simulink model "Energy_based_CBF_shishir"  (R2023b)
settings: Solver=ode5  StartTime=0.0  StopTime=4  FixedStep=0.00001  RelTol=1e-3
settings Model: Creator=amaiani  LastModifiedBy=amaiani

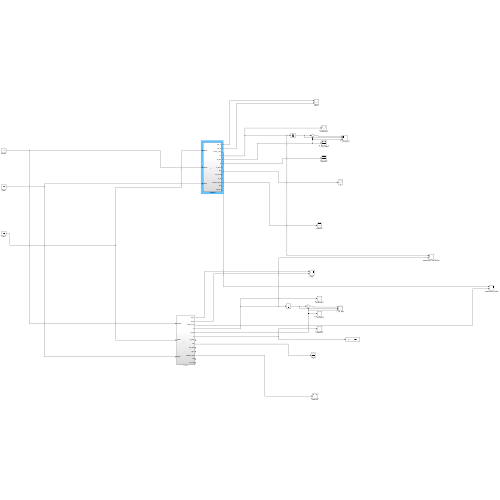
[thumbnail: Simulink's stored preview of the top-level diagram]
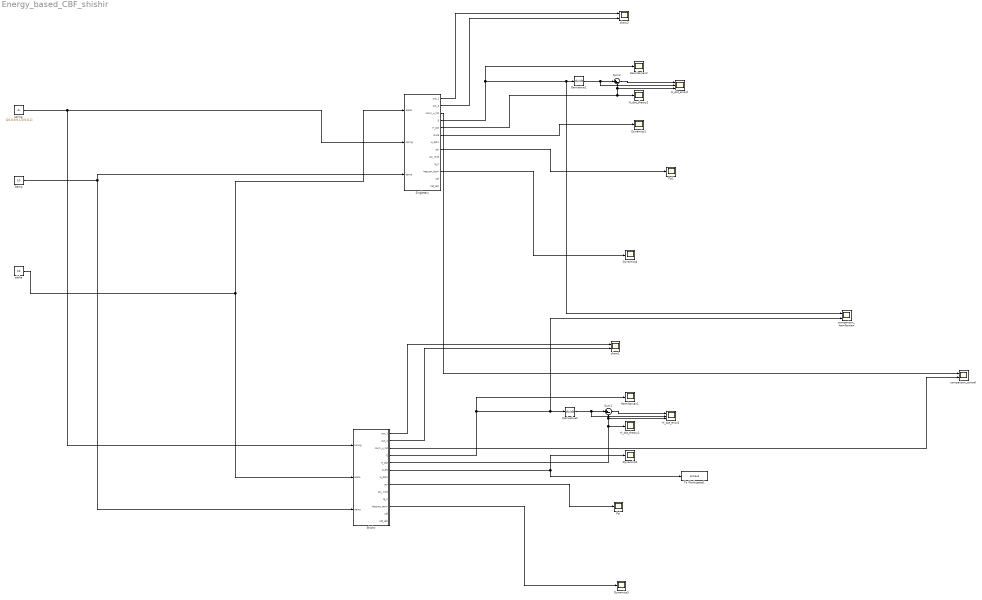
== system Energy_based_CBF_shishir ==
  Damp : Constant  Value=10
  Derivative1 : Derivative
  Derivative2 : Derivative
  Dynamics{1..4} (4 alike) : Scope
  H_dot_error1 : Scope  NumInputPorts=3
  H_dot_error2 : Scope  NumInputPorts=3
  H_dot_theory1 : Scope
  H_dot_theory2 : Scope
  Hamiltonian1 : Scope
  Hamiltonian2 : Scope
  Psi : Scope
  Psi1 : Scope
  Shishir : Subsystem
  Singletary : Subsystem
  Sum1 : Sum  Inputs=|+-
  Sum2 : Sum  Inputs=|+-
  To Workspace1 : ToWorkspace  VariableName=simout  SampleTime=-1
  alpha : Constant  Value=10
  comparison_control : Scope  NumInputPorts=2
  comparison_hamiltonian : Scope  NumInputPorts=2
  skew1 : Scope  NumInputPorts=2
  skew2 : Scope  NumInputPorts=2
  spring : Constant  Value=[10,0,0;0,1,0;0,0,1]
  wires:
  Derivative2/1 -> H_dot_error1/2, Sum1/1
  Sum1/1 -> H_dot_error1/1
  alpha/1 -> Singletary/1(alpha), Shishir/2(alpha)
  Shishir/5(H_dot) -> H_dot_theory1/1, H_dot_error1/3, Sum1/2
  Shishir/4(E) -> Derivative2/1, comparison_hamiltonian/2, Hamiltonian1/1
  Shishir/1(out_1) -> skew1/1
  Shishir/2(out_2) -> skew1/2
  Shishir/3(norm_u_tot) -> comparison_control/2
  Shishir/6(Out6) -> Dynamics2/1, To Workspace1/1
  Shishir/11(hessian_term) -> Dynamics3/1
  Derivative1/1 -> H_dot_error2/2, Sum2/1
  Singletary/1(out_1) -> skew2/1
  Singletary/5(H_dot) -> H_dot_theory2/1, H_dot_error2/3, Sum2/2
  Damp/1 -> Singletary/3(damp), Shishir/3(damp)
  Singletary/2(out_2) -> skew2/2
  Singletary/4(E) -> comparison_hamiltonian/1, Derivative1/1, Hamiltonian2/1
  Sum2/1 -> H_dot_error2/1
  Singletary/3(norm_u_tot) -> comparison_control/1
  Singletary/11(hessian_term) -> Dynamics4/1
  Singletary/6(Out6) -> Dynamics1/1
  spring/1 -> Singletary/2(spring), Shishir/1(spring)
  Shishir/8(psi) -> Psi/1
  Singletary/8(psi) -> Psi1/1

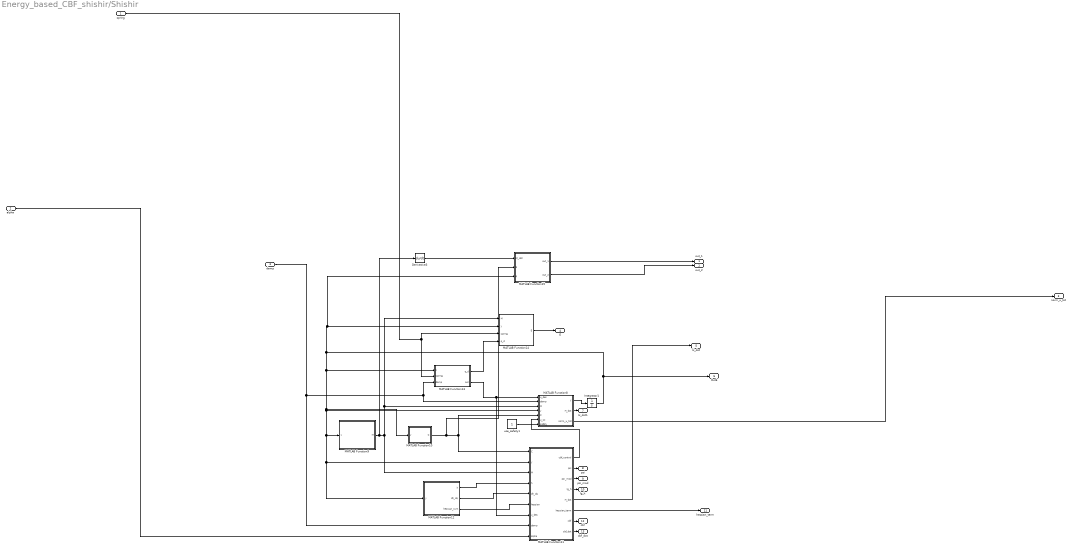
== system Energy_based_CBF_shishir/Shishir ==
  spring : Inport
  alpha : Inport  Port=2
  damp : Inport  Port=3
  Derivative3 : Derivative
  Integrator1 : Integrator  InitialCondition=[0;0;0;0;0;0]
  MATLAB Function10 : MATLAB Function  StartFcn=|  TreatAsAtomicUnit=on
      | % Define numerical values for the parameters
      | xc = 2.5;
      | yc = 2;
      | r = 1;
      | gamma = 2;
      | alpha = 20;
      | 
      | 
      | m1 = 1;
      | m2 = 1;
      | m3 = 1;
      | 
      | 
      | l1 = 1;
      | l2 = 1;
      | l3 = 1;
  MATLAB Function11 : MATLAB Function  TreatAsAtomicUnit=on
  MATLAB Function12 : MATLAB Function  TreatAsAtomicUnit=on
  MATLAB Function13 : MATLAB Function  TreatAsAtomicUnit=on
  MATLAB Function14 : MATLAB Function  TreatAsAtomicUnit=on
  MATLAB Function15 : MATLAB Function  StartFcn=|  TreatAsAtomicUnit=on
      | % Define numerical values for the parameters
      | xc = 2.5;
      | yc = 2;
      | r = 1;
      | gamma = 2;
      | alpha = 20;
      | 
      | 
      | m1 = 1;
      | m2 = 1;
      | m3 = 1;
      | 
      | 
      | l1 = 1;
      | l2 = 1;
      | l3 = 1;
  MATLAB Function8 : MATLAB Function  TreatAsAtomicUnit=on
  MATLAB Function9 : MATLAB Function  StartFcn=|  TreatAsAtomicUnit=on
      | % Define numerical values for the parameters
      | xc = 2.5;
      | yc = 2;
      | r = 1;
      | gamma = 2;
      | alpha = 20;
      | 
      | 
      | m1 = 1;
      | m2 = 1;
      | m3 = 1;
      | 
      | 
      | l1 = 1;
      | l2 = 1;
      | l3 = 1;
  use_safety1 : Constant
  out_1 : Outport
  out_2 : Outport  Port=2
  norm_u_tot : Outport  Port=3
  E : Outport  Port=4
  H_dot : Outport  Port=5
  Out6 : Outport  Port=6
  H_dot1 : Outport  Port=7
  psi : Outport  Port=8
  psi_mod : Outport  Port=9
  lg_h : Outport  Port=10
  hessian_term : Outport  Port=11
  cbf : Outport  Port=12
  cbf_dot : Outport  Port=13
  wires:
  MATLAB Function11/2(psi) -> psi/1
  MATLAB Function11/4(lg_h) -> lg_h/1
  MATLAB Function11/7(cbf) -> cbf/1
  MATLAB Function8/2(H_dot) -> H_dot1/1
  MATLAB Function11/5(H_dot) -> H_dot/1
  MATLAB Function11/6(hessian_term) -> hessian_term/1
  MATLAB Function14/1(E) -> E/1
  MATLAB Function8/3(norm_u_tot) -> norm_u_tot/1
  MATLAB Function12/3(hessian_sym) -> MATLAB Function11/6(hessian)
  Derivative3/1 -> MATLAB Function15/1(M_dot)
  MATLAB Function12/1(h) -> MATLAB Function11/4(h)
  MATLAB Function8/1(y) -> Integrator1/1
  MATLAB Function11/3(psi_mod) -> psi_mod/1
  alpha/1 -> MATLAB Function11/9(alpha)
  spring/1 -> MATLAB Function13/2(spring), MATLAB Function14/3(spring)
  MATLAB Function10/1(C) -> MATLAB Function8/5(C), MATLAB Function11/1(C), MATLAB Function15/2(S)
  MATLAB Function13/1(q_d) -> MATLAB Function14/4(q_d)
  MATLAB Function11/1(cbf_control) -> MATLAB Function8/6(u_sc)
  MATLAB Function15/2(out_2) -> out_2/1
  Integrator1/1 -> Out6/1, MATLAB Function15/3(q), MATLAB Function14/2(y), MATLAB Function13/1(y), MATLAB Function10/1(y), MATLAB Function12/1(y), MATLAB Function11/2(y), MATLAB Function9/1(y), MATLAB Function8/4("y ")
  MATLAB Function15/1(out_1) -> out_1/1
  damp/1 -> MATLAB Function11/8(damp), MATLAB Function8/2(damp), MATLAB Function13/3(damp)
  MATLAB Function12/2(dh_dq) -> MATLAB Function11/5(dh_dq)
  MATLAB Function13/2(out) -> MATLAB Function11/7(u_des), MATLAB Function8/1(u_des)
  MATLAB Function11/8(cbf_dot) -> cbf_dot/1
  use_safety1/1 -> MATLAB Function8/7(safety)
  MATLAB Function9/1(M) -> Derivative3/1, MATLAB Function14/1(M), MATLAB Function8/3(M), MATLAB Function11/3(M)

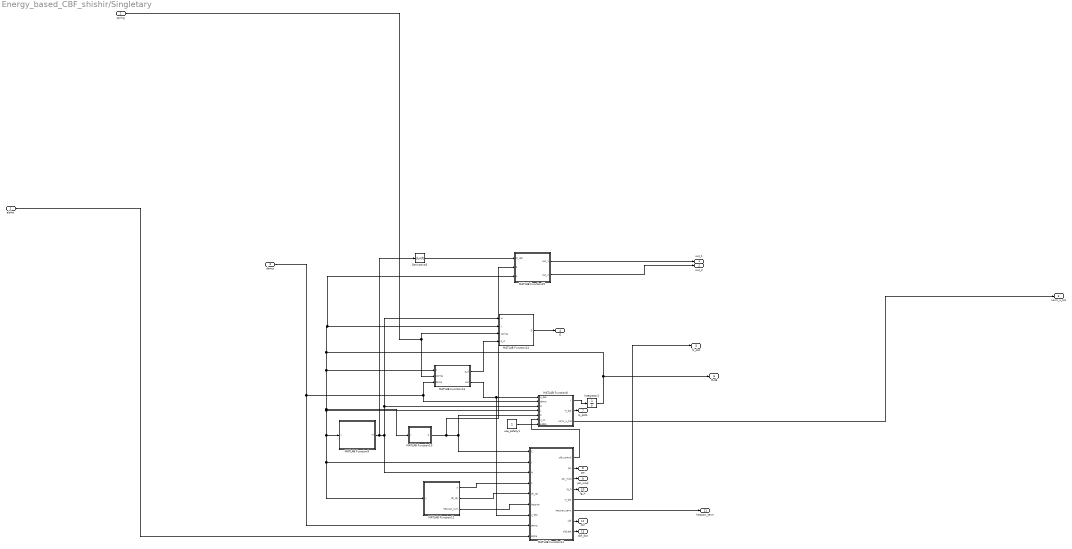
== system Energy_based_CBF_shishir/Singletary ==
  alpha : Inport
  spring : Inport  Port=2
  damp : Inport  Port=3
  Derivative3 : Derivative
  Integrator1 : Integrator  InitialCondition=[0;0;0;0;0;0]
  MATLAB Function10 : MATLAB Function  StartFcn=|  TreatAsAtomicUnit=on
      | % Define numerical values for the parameters
      | xc = 2.5;
      | yc = 2;
      | r = 1;
      | gamma = 2;
      | alpha = 20;
      | 
      | 
      | m1 = 1;
      | m2 = 1;
      | m3 = 1;
      | 
      | 
      | l1 = 1;
      | l2 = 1;
      | l3 = 1;
  MATLAB Function11 : MATLAB Function  TreatAsAtomicUnit=on
  MATLAB Function12 : MATLAB Function  TreatAsAtomicUnit=on
  MATLAB Function13 : MATLAB Function  TreatAsAtomicUnit=on
  MATLAB Function14 : MATLAB Function  TreatAsAtomicUnit=on
  MATLAB Function15 : MATLAB Function  StartFcn=|  TreatAsAtomicUnit=on
      | % Define numerical values for the parameters
      | xc = 2.5;
      | yc = 2;
      | r = 1;
      | gamma = 2;
      | alpha = 20;
      | 
      | 
      | m1 = 1;
      | m2 = 1;
      | m3 = 1;
      | 
      | 
      | l1 = 1;
      | l2 = 1;
      | l3 = 1;
  MATLAB Function8 : MATLAB Function  TreatAsAtomicUnit=on
  MATLAB Function9 : MATLAB Function  StartFcn=|  TreatAsAtomicUnit=on
      | % Define numerical values for the parameters
      | xc = 2.5;
      | yc = 2;
      | r = 1;
      | gamma = 2;
      | alpha = 20;
      | 
      | 
      | m1 = 1;
      | m2 = 1;
      | m3 = 1;
      | 
      | 
      | l1 = 1;
      | l2 = 1;
      | l3 = 1;
  use_safety1 : Constant
  out_1 : Outport
  out_2 : Outport  Port=2
  norm_u_tot : Outport  Port=3
  E : Outport  Port=4
  H_dot : Outport  Port=5
  Out6 : Outport  Port=6
  H_dot1 : Outport  Port=7
  psi : Outport  Port=8
  psi_mod : Outport  Port=9
  lg_h : Outport  Port=10
  hessian_term : Outport  Port=11
  cbf : Outport  Port=12
  cbf_dot : Outport  Port=13
  wires:
  MATLAB Function11/2(psi) -> psi/1
  MATLAB Function11/4(lg_h) -> lg_h/1
  MATLAB Function11/7(cbf) -> cbf/1
  MATLAB Function8/2(H_dot) -> H_dot1/1
  MATLAB Function11/5(H_dot) -> H_dot/1
  MATLAB Function11/6(hessian_term) -> hessian_term/1
  MATLAB Function14/1(E) -> E/1
  MATLAB Function8/3(norm_u_tot) -> norm_u_tot/1
  MATLAB Function12/3(hessian_sym) -> MATLAB Function11/6(hessian)
  Derivative3/1 -> MATLAB Function15/1(M_dot)
  MATLAB Function12/1(h) -> MATLAB Function11/4(h)
  MATLAB Function8/1(y) -> Integrator1/1
  MATLAB Function11/3(psi_mod) -> psi_mod/1
  alpha/1 -> MATLAB Function11/9(alpha)
  spring/1 -> MATLAB Function13/2(spring), MATLAB Function14/3(spring)
  MATLAB Function10/1(C) -> MATLAB Function8/5(C), MATLAB Function11/1(C), MATLAB Function15/2(S)
  MATLAB Function13/1(q_d) -> MATLAB Function14/4(q_d)
  MATLAB Function11/1(cbf_control) -> MATLAB Function8/6(u_sc)
  MATLAB Function15/2(out_2) -> out_2/1
  Integrator1/1 -> Out6/1, MATLAB Function15/3(q), MATLAB Function14/2(y), MATLAB Function13/1(y), MATLAB Function10/1(y), MATLAB Function12/1(y), MATLAB Function11/2(y), MATLAB Function9/1(y), MATLAB Function8/4("y ")
  MATLAB Function15/1(out_1) -> out_1/1
  damp/1 -> MATLAB Function11/8(damp), MATLAB Function8/2(damp), MATLAB Function13/3(damp)
  MATLAB Function12/2(dh_dq) -> MATLAB Function11/5(dh_dq)
  MATLAB Function13/2(out) -> MATLAB Function11/7(u_des), MATLAB Function8/1(u_des)
  MATLAB Function11/8(cbf_dot) -> cbf_dot/1
  use_safety1/1 -> MATLAB Function8/7(safety)
  MATLAB Function9/1(M) -> Derivative3/1, MATLAB Function14/1(M), MATLAB Function8/3(M), MATLAB Function11/3(M)

== matlab function Energy_based_CBF_shishir/Singletary/MATLAB Function9 ==
  data: y input; M output
function M = inertia_M(y)

    q1 = y(1);
    q2 = y(2);
    q3 = y(3);

    M  = [        cos(q2 + q3) + 3*cos(q2) + cos(q3) + 4, cos(q2 + q3)/2 + (3*cos(q2))/2 + cos(q3) + 5/3, cos(q2 + q3)/2 + cos(q3)/2 + 1/3;
cos(q2 + q3)/2 + (3*cos(q2))/2 + cos(q3) + 5/3,                                  cos(q3) + 5/3,                  cos(q3)/2 + 1/3;
              cos(q2 + q3)/2 + cos(q3)/2 + 1/3,                                cos(q3)/2 + 1/3,                              1/3];

== matlab function Energy_based_CBF_shishir/Shishir/MATLAB Function10 ==
  data: y input; C output
function C = coriolis(y)

    q1 = y(1);
    q2 = y(2);
    q3 = y(3);
    dq1 = y(4);
    dq2 = y(5);
    dq3 = y(6);


    C = [- dq2*(sin(q2 + q3)/2 + (3*sin(q2))/2) - dq3*(sin(q2 + q3)/2 + sin(q3)/2), - dq1*(sin(q2 + q3)/2 + (3*sin(q2))/2) - dq2*(sin(q2 + q3)/2 + (3*sin(q2))/2) - dq3*(sin(q2 + q3)/2 + sin(q3)/2), - dq1*(sin(q2 + q3)/2 + sin(q3)/2) - dq2*(sin(q2 + q3)/2 + sin(q3)/2) - dq3*(sin(q2 + q3)/2 + sin(q3)/2);
                dq1*(sin(q2 + q3)/2 + (3*sin(q2))/2) - (dq3*sin(q3))/2,                                                                                                 -(dq3*sin(q3))/2,                                                    - (dq1*sin(q3))/2 - (dq2*sin(q3))/2 - (dq3*sin(q3))/2;
                       dq1*(sin(q2 + q3)/2 + sin(q3)/2) + (dq2*sin(q3))/2,                                                                                (dq1*sin(q3))/2 + (dq2*sin(q3))/2,                                                                                                        0];

== matlab function Energy_based_CBF_shishir/Shishir/MATLAB Function11 ==
  data: C input; y input; cbf_control output; M input; h input; dh_dq input; hessian input; u_des input; psi output; psi_mod output; lg_h output; H_dot output; damp input; hessian_term output; cbf output; cbf_dot output; alpha input

function [cbf_control, psi, psi_mod,lg_h, H_dot, hessian_term, cbf, cbf_dot]= CBF(C, y, M, h, dh_dq, hessian, u_des, damp, alpha)
% Define numerical values for the parameters
    xc = 2.5;
    yc = 2;
    r = 1;
    gamma = 2;

    
    m1 = 1;
    m2 = 1;
    m3 = 1;
    
    l1 = 1;
    l2 = 1;
    l3 = 1;
    
    q = reshape(y(1:3),[3,1]);
    dq = reshape(y(4:6),[3,1]);
    dh_dq = reshape(dh_dq,[1,3]);

    shishir = 1;

    if shishir == 1

    
        
        KE = 0.5 * dq' * M * dq;
        cbf = 1/h + KE/(1+KE);
        lg_h = zeros(1,3);
        cbf_dot_prior = - 1/h^2 * (dh_dq * dq)- 1/(1+KE)^2 * dq' * damp * dq;
        psi = cbf_dot_prior - gamma .* h;
        if psi>0
            lg_h = dq'/(1+KE)^2;
            cbf_control =  -lg_h' /(lg_h*lg_h')  .* psi;
        else
            cbf_control = zeros(3,1);
        end
        cbf_dot =  - 1/h^2 * (dh_dq * dq)- 1/(1+KE)^2 * dq' * damp * dq + lg_h * cbf_control;
        psi_mod = cbf_dot - gamma .* h;

        H_dot = dq' * cbf_control - dq' * damp * dq;


        hessian_term = 0;
    
    else
        KE = 0.5 * dq' * M * dq;
        cbf = alpha * h - KE;
        lg_h = zeros(1,3);
        cbf_dot_prior = alpha .* dh_dq * dq - dq' * inv(M) * u_des;
        psi = cbf_dot_prior + gamma .* cbf;
        if psi<0
            lg_h = -dq';
            cbf_control =  dq /(dq'*dq)  .* psi;
        else
            cbf_control = zeros(3,1);
        end
        cbf_dot =  alpha .* dh_dq * dq - dq' * inv(M) * (u_des+cbf_control) ;
        psi_mod = cbf_dot + gamma .* cbf;

        H_dot = dq' * cbf_control - dq' * damp * dq;


        hessian_term = 0;
        
    end
    
end

== matlab function Energy_based_CBF_shishir/Shishir/MATLAB Function12 ==
  data: y input; h output; dh_dq output; hessian_sym output
function [h, dh_dq, hessian_sym] = obstacle(y)
    % Define numerical values for the parameters
    xc = 2.5;
    yc = 2;
    r = 1;

    l1 = 1;
    l2 = 1;
    l3 = 1;
    
    % Compute the end-effector position using forward kinematics
    q1 = y(1);
    q2 = y(2);
    q3 = y(3);
    
    x_ee = l1 * cos(q1) + l2 * cos(q1 + q2) + l3 * cos(q1 + q2 + q3);
    y_ee = l1 * sin(q1) + l2 * sin(q1 + q2) + l3 * sin(q1 + q2 + q3);
    
    % Compute the control barrier function h
    h = (xc - x_ee)^2 + (yc - y_ee)^2 - r^2;
    
    % Define the expressions for dh_dq and hessian_sym
    dh_dq = [2*(cos(q1 + q2 + q3) + cos(q1 + q2) + cos(q1))*(sin(q1 + q2 + q3) + sin(q1 + q2) + sin(q1) - 2) - 2*(sin(q1 + q2 + q3) + sin(q1 + q2) + sin(q1))*(cos(q1 + q2 + q3) + cos(q1 + q2) + cos(q1) - 5/2), 2*(cos(q1 + q2 + q3) + cos(q1 + q2))*(sin(q1 + q2 + q3) + sin(q1 + q2) + sin(q1) - 2) - 2*(sin(q1 + q2 + q3) + sin(q1 + q2))*(cos(q1 + q2 + q3) + cos(q1 + q2) + cos(q1) - 5/2), 2*cos(q1 + q2 + q3)*(sin(q1 + q2 + q3) + sin(q1 + q2) + sin(q1) - 2) - 2*sin(q1 + q2 + q3)*(cos(q1 + q2 + q3) + cos(q1 + q2) + cos(q1) - 5/2)];


    hessian_sym = [                                              2*(cos(q1 + q2 + q3) + cos(q1 + q2) + cos(q1))^2 - 2*(cos(q1 + q2 + q3) + cos(q1 + q2) + cos(q1))*(cos(q1 + q2 + q3) + cos(q1 + q2) + cos(q1) - 5/2) + 2*(sin(q1 + q2 + q3) + sin(q1 + q2) + sin(q1))^2 - 2*(sin(q1 + q2 + q3) + sin(q1 + q2) + sin(q1))*(sin(q1 + q2 + q3) + sin(q1 + q2) + sin(q1) - 2), 2*(cos(q1 + q2 + q3) + cos(q1 + q2))*(cos(q1 + q2 + q3) + cos(q1 + q2) + cos(q1)) - 2*(cos(q1 + q2 + q3) + cos(q1 + q2))*(cos(q1 + q2 + q3) + cos(q1 + q2) + cos(q1) - 5/2) + 2*(sin(q1 + q2 + q3) + sin(q1 + q2))*(sin(q1 + q2 + q3) + sin(q1 + q2) + sin(q1)) - 2*(sin(q1 + q2 + q3) + sin(q1 + q2))*(sin(q1 + q2 + q3) + sin(q1 + q2) + sin(q1) - 2), 2*cos(q1 + q2 + q3)*(cos(q1 + q2 + q3) + cos(q1 + q2) + cos(q1)) - 2*cos(q1 + q2 + q3)*(cos(q1 + q2 + q3) + cos(q1 + q2) + cos(q1) - 5/2) + 2*sin(q1 + q2 + q3)*(sin(q1 + q2 + q3) + sin(q1 + q2) + sin(q1)) - 2*sin(q1 + q2 + q3)*(sin(q1 + q2 + q3) + sin(q1 + q2) + sin(q1) - 2);
        2*(cos(q1 + q2 + q3) + cos(q1 + q2))*(cos(q1 + q2 + q3) + cos(q1 + q2) + cos(q1)) - 2*(cos(q1 + q2 + q3) + cos(q1 + q2))*(cos(q1 + q2 + q3) + cos(q1 + q2) + cos(q1) - 5/2) + 2*(sin(q1 + q2 + q3) + sin(q1 + q2))*(sin(q1 + q2 + q3) + sin(q1 + q2) + sin(q1)) - 2*(sin(q1 + q2 + q3) + sin(q1 + q2))*(sin(q1 + q2 + q3) + sin(q1 + q2) + sin(q1) - 2),                                                                                       2*(cos(q1 + q2 + q3) + cos(q1 + q2))^2 - 2*(cos(q1 + q2 + q3) + cos(q1 + q2))*(cos(q1 + q2 + q3) + cos(q1 + q2) + cos(q1) - 5/2) + 2*(sin(q1 + q2 + q3) + sin(q1 + q2))^2 - 2*(sin(q1 + q2 + q3) + sin(q1 + q2))*(sin(q1 + q2 + q3) + sin(q1 + q2) + sin(q1) - 2),                     2*cos(q1 + q2 + q3)*(cos(q1 + q2 + q3) + cos(q1 + q2)) - 2*cos(q1 + q2 + q3)*(cos(q1 + q2 + q3) + cos(q1 + q2) + cos(q1) - 5/2) - 2*sin(q1 + q2 + q3)*(sin(q1 + q2 + q3) + sin(q1 + q2) + sin(q1) - 2) + 2*sin(q1 + q2 + q3)*(sin(q1 + q2 + q3) + sin(q1 + q2));
                                                                            2*cos(q1 + q2 + q3)*(cos(q1 + q2 + q3) + cos(q1 + q2) + cos(q1)) - 2*cos(q1 + q2 + q3)*(cos(q1 + q2 + q3) + cos(q1 + q2) + cos(q1) - 5/2) + 2*sin(q1 + q2 + q3)*(sin(q1 + q2 + q3) + sin(q1 + q2) + sin(q1)) - 2*sin(q1 + q2 + q3)*(sin(q1 + q2 + q3) + sin(q1 + q2) + sin(q1) - 2),                                                                                         2*cos(q1 + q2 + q3)*(cos(q1 + q2 + q3) + cos(q1 + q2)) - 2*cos(q1 + q2 + q3)*(cos(q1 + q2 + q3) + cos(q1 + q2) + cos(q1) - 5/2) - 2*sin(q1 + q2 + q3)*(sin(q1 + q2 + q3) + sin(q1 + q2) + sin(q1) - 2) + 2*sin(q1 + q2 + q3)*(sin(q1 + q2 + q3) + sin(q1 + q2)),                                                                                       2*cos(q1 + q2 + q3)^2 - 2*cos(q1 + q2 + q3)*(cos(q1 + q2 + q3) + cos(q1 + q2) + cos(q1) - 5/2) + 2*sin(q1 + q2 + q3)^2 - 2*sin(q1 + q2 + q3)*(sin(q1 + q2 + q3) + sin(q1 + q2) + sin(q1) - 2)];
     

    % d = eig(hessian_sym)
    % isposdef = all(d >= 0);
    % 
    % assert(isposdef, 'error hessian');
end

== matlab function Energy_based_CBF_shishir/Shishir/MATLAB Function13 ==
  data: q_d output; y input; spring input; out output; damp input
function [q_d, out] = u_des(y, spring, damp)


    q = reshape(y(1:3),[3,1]);
    dq = reshape(y(4:6),[3,1]);

    q_d = [pi; 0; pi/4];
    
    out =  - damp * dq - spring * (q-q_d);

== matlab function Energy_based_CBF_shishir/Shishir/MATLAB Function14 ==
  data: M input; E output; y input; spring input; q_d input
function E = energy(M,y,spring, q_d)
    q = y(1:3);
    dq = y(4:6);
    

    E = 0.5 * (dq' * M * dq) + 0.5 * (q-q_d)'* spring * (q-q_d);

== matlab function Energy_based_CBF_shishir/Shishir/MATLAB Function15 ==
  data: M_dot input; out_1 output; S input; q input; out_2 output


function [out_1, out_2] = M_dot_coriolis_check(M_dot,S, q)
    dq = reshape(q(4:6),[3,1]);
    
    q1 = q(1);
    q2 = q(2);
    q3 = q(3);
    dq1 = q(4);
    dq2 = q(5);
    dq3 = q(6);

    check = M_dot - 2 * S;


    out_1 = dq' * check * dq;


    M_dot_formula =   [        - dq2*(sin(q2 + q3) + 3*sin(q2)) - dq3*(sin(q2 + q3) + sin(q3)), - dq3*(sin(q2 + q3)/2 + sin(q3)) - dq2*(sin(q2 + q3)/2 + (3*sin(q2))/2), - (dq2*sin(q2 + q3))/2 - dq3*(sin(q2 + q3)/2 + sin(q3)/2);
- dq3*(sin(q2 + q3)/2 + sin(q3)) - dq2*(sin(q2 + q3)/2 + (3*sin(q2))/2),                                                            -dq3*sin(q3),                                          -(dq3*sin(q3))/2;
              - (dq2*sin(q2 + q3))/2 - dq3*(sin(q2 + q3)/2 + sin(q3)/2),                                                        -(dq3*sin(q3))/2,                                                         0];
 

    
    out_2 = dq' * (M_dot_formula - 2 * S) * dq;
end

== matlab function Energy_based_CBF_shishir/Shishir/MATLAB Function8 ==
  data: u_des input; damp input; M input; y input; y output; C input; H_dot output; u_sc input; safety input; norm_u_tot output
function [y,H_dot,norm_u_tot]= dynamics(u_des, damp , M,y, C, u_sc, safety)
    
    q = reshape(y(1:3),[3,1]);
    dq = reshape(y(4:6),[3,1]);



    [~, p] = chol(M);
    decision = (p == 0);

    assert(decision, 'Inertia matrix is not positive definite');
    
    u_tot = u_des + safety * u_sc;
    norm_u_tot=norm(u_tot);
    ddq = inv(M) * (u_tot - C * dq ); % + u_sc

    H_dot = - dq' * damp * dq;

    y = [dq; ddq];

== matlab function Energy_based_CBF_shishir/Shishir/MATLAB Function9 ==
  data: y input; M output
function M = inertia_M(y)

    q1 = y(1);
    q2 = y(2);
    q3 = y(3);

    M  = [        cos(q2 + q3) + 3*cos(q2) + cos(q3) + 4, cos(q2 + q3)/2 + (3*cos(q2))/2 + cos(q3) + 5/3, cos(q2 + q3)/2 + cos(q3)/2 + 1/3;
cos(q2 + q3)/2 + (3*cos(q2))/2 + cos(q3) + 5/3,                                  cos(q3) + 5/3,                  cos(q3)/2 + 1/3;
              cos(q2 + q3)/2 + cos(q3)/2 + 1/3,                                cos(q3)/2 + 1/3,                              1/3];

== matlab function Energy_based_CBF_shishir/Singletary/MATLAB Function10 ==
  data: y input; C output
function C = coriolis(y)

    q1 = y(1);
    q2 = y(2);
    q3 = y(3);
    dq1 = y(4);
    dq2 = y(5);
    dq3 = y(6);


    C = [- dq2*(sin(q2 + q3)/2 + (3*sin(q2))/2) - dq3*(sin(q2 + q3)/2 + sin(q3)/2), - dq1*(sin(q2 + q3)/2 + (3*sin(q2))/2) - dq2*(sin(q2 + q3)/2 + (3*sin(q2))/2) - dq3*(sin(q2 + q3)/2 + sin(q3)/2), - dq1*(sin(q2 + q3)/2 + sin(q3)/2) - dq2*(sin(q2 + q3)/2 + sin(q3)/2) - dq3*(sin(q2 + q3)/2 + sin(q3)/2);
                dq1*(sin(q2 + q3)/2 + (3*sin(q2))/2) - (dq3*sin(q3))/2,                                                                                                 -(dq3*sin(q3))/2,                                                    - (dq1*sin(q3))/2 - (dq2*sin(q3))/2 - (dq3*sin(q3))/2;
                       dq1*(sin(q2 + q3)/2 + sin(q3)/2) + (dq2*sin(q3))/2,                                                                                (dq1*sin(q3))/2 + (dq2*sin(q3))/2,                                                                                                        0];

== matlab function Energy_based_CBF_shishir/Singletary/MATLAB Function11 ==
  data: C input; y input; cbf_control output; M input; h input; dh_dq input; hessian input; u_des input; psi output; psi_mod output; lg_h output; H_dot output; damp input; hessian_term output; cbf output; cbf_dot output; alpha input

function [cbf_control, psi, psi_mod,lg_h, H_dot, hessian_term, cbf, cbf_dot]= CBF(C, y, M, h, dh_dq, hessian, u_des, damp, alpha)
% Define numerical values for the parameters
    xc = 2.5;
    yc = 2;
    r = 1;
    gamma = 2;

    
    m1 = 1;
    m2 = 1;
    m3 = 1;
    
    l1 = 1;
    l2 = 1;
    l3 = 1;
    
    q = reshape(y(1:3),[3,1]);
    dq = reshape(y(4:6),[3,1]);
    dh_dq = reshape(dh_dq,[1,3]);

    shishir = 0;

    if shishir == 1

    
        
        KE = 0.5 * dq' * M * dq;
        cbf = 1/h + KE/(1+KE);
        lg_h = zeros(1,3);
        cbf_dot_prior = - 1/h^2 * (dh_dq * dq)- 1/(1+KE)^2 * dq' * damp * dq;
        psi = cbf_dot_prior - gamma .* h;
        if psi>0
            lg_h = dq'/(1+KE)^2;
            cbf_control =  -lg_h' /(lg_h*lg_h')  .* psi;
        else
            cbf_control = zeros(3,1);
        end
        cbf_dot =  - 1/h^2 * (dh_dq * dq)- 1/(1+KE)^2 * dq' * damp * dq + lg_h * cbf_control;
        psi_mod = cbf_dot - gamma .* h;

        H_dot = dq' * cbf_control - dq' * damp * dq;


        hessian_term = 0;
    
    else
        KE = 0.5 * dq' * M * dq;
        cbf = alpha * h - KE;
        lg_h = zeros(1,3);
        cbf_dot_prior = alpha .* dh_dq * dq - dq' * u_des;
        psi = cbf_dot_prior + gamma .* cbf;
        if psi<0
            lg_h = -dq';
            cbf_control =  dq /(dq'*dq)  .* psi;
        else
            cbf_control = zeros(3,1);
        end
        cbf_dot =  alpha .* dh_dq * dq - dq' * (u_des+cbf_control) ;
        psi_mod = cbf_dot + gamma .* cbf;

        H_dot = dq' * cbf_control - dq' * damp * dq;


        hessian_term = 0;
        
    end
    
end

== matlab function Energy_based_CBF_shishir/Singletary/MATLAB Function12 ==
  data: y input; h output; dh_dq output; hessian_sym output
function [h, dh_dq, hessian_sym] = obstacle(y)
    % Define numerical values for the parameters
    xc = 2.5;
    yc = 2;
    r = 1;

    l1 = 1;
    l2 = 1;
    l3 = 1;
    
    % Compute the end-effector position using forward kinematics
    q1 = y(1);
    q2 = y(2);
    q3 = y(3);
    
    x_ee = l1 * cos(q1) + l2 * cos(q1 + q2) + l3 * cos(q1 + q2 + q3);
    y_ee = l1 * sin(q1) + l2 * sin(q1 + q2) + l3 * sin(q1 + q2 + q3);
    
    % Compute the control barrier function h
    h = (xc - x_ee)^2 + (yc - y_ee)^2 - r^2;
    
    % Define the expressions for dh_dq and hessian_sym
    dh_dq = [2*(cos(q1 + q2 + q3) + cos(q1 + q2) + cos(q1))*(sin(q1 + q2 + q3) + sin(q1 + q2) + sin(q1) - 2) - 2*(sin(q1 + q2 + q3) + sin(q1 + q2) + sin(q1))*(cos(q1 + q2 + q3) + cos(q1 + q2) + cos(q1) - 5/2), 2*(cos(q1 + q2 + q3) + cos(q1 + q2))*(sin(q1 + q2 + q3) + sin(q1 + q2) + sin(q1) - 2) - 2*(sin(q1 + q2 + q3) + sin(q1 + q2))*(cos(q1 + q2 + q3) + cos(q1 + q2) + cos(q1) - 5/2), 2*cos(q1 + q2 + q3)*(sin(q1 + q2 + q3) + sin(q1 + q2) + sin(q1) - 2) - 2*sin(q1 + q2 + q3)*(cos(q1 + q2 + q3) + cos(q1 + q2) + cos(q1) - 5/2)];


    hessian_sym = [                                              2*(cos(q1 + q2 + q3) + cos(q1 + q2) + cos(q1))^2 - 2*(cos(q1 + q2 + q3) + cos(q1 + q2) + cos(q1))*(cos(q1 + q2 + q3) + cos(q1 + q2) + cos(q1) - 5/2) + 2*(sin(q1 + q2 + q3) + sin(q1 + q2) + sin(q1))^2 - 2*(sin(q1 + q2 + q3) + sin(q1 + q2) + sin(q1))*(sin(q1 + q2 + q3) + sin(q1 + q2) + sin(q1) - 2), 2*(cos(q1 + q2 + q3) + cos(q1 + q2))*(cos(q1 + q2 + q3) + cos(q1 + q2) + cos(q1)) - 2*(cos(q1 + q2 + q3) + cos(q1 + q2))*(cos(q1 + q2 + q3) + cos(q1 + q2) + cos(q1) - 5/2) + 2*(sin(q1 + q2 + q3) + sin(q1 + q2))*(sin(q1 + q2 + q3) + sin(q1 + q2) + sin(q1)) - 2*(sin(q1 + q2 + q3) + sin(q1 + q2))*(sin(q1 + q2 + q3) + sin(q1 + q2) + sin(q1) - 2), 2*cos(q1 + q2 + q3)*(cos(q1 + q2 + q3) + cos(q1 + q2) + cos(q1)) - 2*cos(q1 + q2 + q3)*(cos(q1 + q2 + q3) + cos(q1 + q2) + cos(q1) - 5/2) + 2*sin(q1 + q2 + q3)*(sin(q1 + q2 + q3) + sin(q1 + q2) + sin(q1)) - 2*sin(q1 + q2 + q3)*(sin(q1 + q2 + q3) + sin(q1 + q2) + sin(q1) - 2);
        2*(cos(q1 + q2 + q3) + cos(q1 + q2))*(cos(q1 + q2 + q3) + cos(q1 + q2) + cos(q1)) - 2*(cos(q1 + q2 + q3) + cos(q1 + q2))*(cos(q1 + q2 + q3) + cos(q1 + q2) + cos(q1) - 5/2) + 2*(sin(q1 + q2 + q3) + sin(q1 + q2))*(sin(q1 + q2 + q3) + sin(q1 + q2) + sin(q1)) - 2*(sin(q1 + q2 + q3) + sin(q1 + q2))*(sin(q1 + q2 + q3) + sin(q1 + q2) + sin(q1) - 2),                                                                                       2*(cos(q1 + q2 + q3) + cos(q1 + q2))^2 - 2*(cos(q1 + q2 + q3) + cos(q1 + q2))*(cos(q1 + q2 + q3) + cos(q1 + q2) + cos(q1) - 5/2) + 2*(sin(q1 + q2 + q3) + sin(q1 + q2))^2 - 2*(sin(q1 + q2 + q3) + sin(q1 + q2))*(sin(q1 + q2 + q3) + sin(q1 + q2) + sin(q1) - 2),                     2*cos(q1 + q2 + q3)*(cos(q1 + q2 + q3) + cos(q1 + q2)) - 2*cos(q1 + q2 + q3)*(cos(q1 + q2 + q3) + cos(q1 + q2) + cos(q1) - 5/2) - 2*sin(q1 + q2 + q3)*(sin(q1 + q2 + q3) + sin(q1 + q2) + sin(q1) - 2) + 2*sin(q1 + q2 + q3)*(sin(q1 + q2 + q3) + sin(q1 + q2));
                                                                            2*cos(q1 + q2 + q3)*(cos(q1 + q2 + q3) + cos(q1 + q2) + cos(q1)) - 2*cos(q1 + q2 + q3)*(cos(q1 + q2 + q3) + cos(q1 + q2) + cos(q1) - 5/2) + 2*sin(q1 + q2 + q3)*(sin(q1 + q2 + q3) + sin(q1 + q2) + sin(q1)) - 2*sin(q1 + q2 + q3)*(sin(q1 + q2 + q3) + sin(q1 + q2) + sin(q1) - 2),                                                                                         2*cos(q1 + q2 + q3)*(cos(q1 + q2 + q3) + cos(q1 + q2)) - 2*cos(q1 + q2 + q3)*(cos(q1 + q2 + q3) + cos(q1 + q2) + cos(q1) - 5/2) - 2*sin(q1 + q2 + q3)*(sin(q1 + q2 + q3) + sin(q1 + q2) + sin(q1) - 2) + 2*sin(q1 + q2 + q3)*(sin(q1 + q2 + q3) + sin(q1 + q2)),                                                                                       2*cos(q1 + q2 + q3)^2 - 2*cos(q1 + q2 + q3)*(cos(q1 + q2 + q3) + cos(q1 + q2) + cos(q1) - 5/2) + 2*sin(q1 + q2 + q3)^2 - 2*sin(q1 + q2 + q3)*(sin(q1 + q2 + q3) + sin(q1 + q2) + sin(q1) - 2)];
     

    % d = eig(hessian_sym)
    % isposdef = all(d >= 0);
    % 
    % assert(isposdef, 'error hessian');
end

== matlab function Energy_based_CBF_shishir/Singletary/MATLAB Function13 ==
  data: q_d output; y input; spring input; out output; damp input
function [q_d, out] = u_des(y, spring, damp)


    q = reshape(y(1:3),[3,1]);
    dq = reshape(y(4:6),[3,1]);

    q_d = [pi; 0; pi/4];
    
    out =  - damp * dq - spring * (q-q_d);

== matlab function Energy_based_CBF_shishir/Singletary/MATLAB Function14 ==
  data: M input; E output; y input; spring input; q_d input
function E = energy(M,y,spring, q_d)
    q = y(1:3);
    dq = y(4:6);
    

    E = 0.5 * (dq' * M * dq) + 0.5 * (q-q_d)' *spring* (q-q_d);

== matlab function Energy_based_CBF_shishir/Singletary/MATLAB Function15 ==
  data: M_dot input; out_1 output; S input; q input; out_2 output


function [out_1, out_2] = M_dot_coriolis_check(M_dot,S, q)
    dq = reshape(q(4:6),[3,1]);
    
    q1 = q(1);
    q2 = q(2);
    q3 = q(3);
    dq1 = q(4);
    dq2 = q(5);
    dq3 = q(6);

    check = M_dot - 2 * S;


    out_1 = dq' * check * dq;


    M_dot_formula =   [        - dq2*(sin(q2 + q3) + 3*sin(q2)) - dq3*(sin(q2 + q3) + sin(q3)), - dq3*(sin(q2 + q3)/2 + sin(q3)) - dq2*(sin(q2 + q3)/2 + (3*sin(q2))/2), - (dq2*sin(q2 + q3))/2 - dq3*(sin(q2 + q3)/2 + sin(q3)/2);
- dq3*(sin(q2 + q3)/2 + sin(q3)) - dq2*(sin(q2 + q3)/2 + (3*sin(q2))/2),                                                            -dq3*sin(q3),                                          -(dq3*sin(q3))/2;
              - (dq2*sin(q2 + q3))/2 - dq3*(sin(q2 + q3)/2 + sin(q3)/2),                                                        -(dq3*sin(q3))/2,                                                         0];
 

    
    out_2 = dq' * (M_dot_formula - 2 * S) * dq;
end

== matlab function Energy_based_CBF_shishir/Singletary/MATLAB Function8 ==
  data: u_des input; damp input; M input; y input; y output; C input; H_dot output; u_sc input; safety input; norm_u_tot output
function [y,H_dot,norm_u_tot]= dynamics(u_des, damp , M,y, C, u_sc, safety)
    
    q = reshape(y(1:3),[3,1]);
    dq = reshape(y(4:6),[3,1]);



    [~, p] = chol(M);
    decision = (p == 0);

    assert(decision, 'Inertia matrix is not positive definite');
    
    u_tot = u_des + safety * u_sc;
    norm_u_tot=norm(u_tot);
    ddq = inv(M) * (u_tot - C * dq ); % + u_sc

    H_dot = - dq' * damp * dq;

    y = [dq; ddq];
